simulink model "eAgriBot_V4"  (R2022b)
settings: Solver=ode3  StartTime=0.0  StopTime=t_sim  FixedStep=step_size  RelTol=1e-3
values from neighbouring files (symbols this model uses):
  accel = 0.1*9.81    (= 0.981)    [Run_eAgriBot_V4.m]
  B_tines = 5    [Run_eAgriBot_V4.m]
  brake_bias = 1    [Run_eAgriBot_V4.m]
  c = 6100    [Run_eAgriBot_V4.m]
  decel = 0.15*9.81    (= 1.4715)    [Run_eAgriBot_V4.m]
  decel_begin_dist = total_dist_target    (= 100)    [Run_eAgriBot_V4.m]
  drivetype = 3    [Run_eAgriBot_V4.m]
  effmap = [0.5 0.586 0.723 0.778 0.614 0.604 0.6 0.584 0.709 0.658 0.586 0.688 ... (121 elements, 11x11)]    [EM_effmap_generic.mat]
  end_delay = 4    [Run_eAgriBot_V4.m]
  F_tines = 5    [Run_eAgriBot_V4.m]
  Fb_max = m*g    (= 5101.2)    [Run_eAgriBot_V4.m]
  FT_c_x_rel = l_f    (= 0.645)    [Run_eAgriBot_V4.m]
  FT_c_z_rel = R_u-h_CoG    (= -0.2825)    [Run_eAgriBot_V4.m]
  g = 9.81    [Run_eAgriBot_V4.m]
  gb_eff = 0.98    [Run_eAgriBot_V4.m]
  ground_coh = c*ones(length(ground_points),1)    [Run_eAgriBot_V4.m]
  ground_dens = gamma_s*ones(length(ground_points),1)    [Run_eAgriBot_V4.m]
  ground_height = zeros(length(ground_points),1)    [Run_eAgriBot_V4.m]
  ground_kxy = k_xy*ones(length(ground_points),1)    [Run_eAgriBot_V4.m]
  ground_res = 0.01    [Run_eAgriBot_V4.m]
  Har_back_tip_x_rel = Har_back_top_x_rel+Har_tine_length*cos(Har_angle)    [Run_eAgriBot_V4.m]
  Har_back_tip_z_rel = abs(Hook_z_rel)-h_CoG-Har_tine_depth    [Run_eAgriBot_V4.m]
  Har_back_top_x_rel = -2.0    (= -2)    [Run_eAgriBot_V4.m]
  Har_back_top_z_rel = Har_back_tip_z_rel+Har_tine_length*sin(Har_angle)    [Run_eAgriBot_V4.m]
  Har_front_tip_x_rel = Har_front_top_x_rel+Har_tine_length*cos(Har_angle)    [Run_eAgriBot_V4.m]
  Har_front_tip_z_rel = abs(Hook_z_rel)-h_CoG-Har_tine_depth    [Run_eAgriBot_V4.m]
  Har_front_top_x_rel = -1.2    [Run_eAgriBot_V4.m]
  Har_front_top_z_rel = Har_front_tip_z_rel+Har_tine_length*sin(Har_angle)    [Run_eAgriBot_V4.m]
  Har_tine_length = 0.25    [Run_eAgriBot_V4.m]
  Har_tine_width = 0.02    [Run_eAgriBot_V4.m]
  Har_tire_rad = 0.5842/2    (= 0.2921)    [Run_eAgriBot_V4.m]
  Har_tire_x_rel = -1.5    [Run_eAgriBot_V4.m]
  Har_tire_z_rel = abs(Hook_z_rel)-h_CoG+Har_tire_rad    [Run_eAgriBot_V4.m]
  Hook_x_rel = l_f-l-0.4    (= -1.045)    [Run_eAgriBot_V4.m]
  Hook_z_rel = -0.3    [Run_eAgriBot_V4.m]
  i_front = 17.9542    [Run_eAgriBot_V4.m]
  I_gain = 0.0    (= 0)    [Run_eAgriBot_V4.m]
  i_rear = 17.9542    [Run_eAgriBot_V4.m]
  I_y = 150    [Run_eAgriBot_V4.m]
  I_y_tool = 20    [Run_eAgriBot_V4.m]
  index_init = round(FT_init_exit_x/ground_res)+1    [Run_eAgriBot_V4.m]
  init_CoG_height = h_CoG-0.001    (= 0.599)    [Run_eAgriBot_V4.m]
  init_CoG_v_z = 0    [Run_eAgriBot_V4.m]
  init_omega = 0    [Run_eAgriBot_V4.m]
  init_theta = 0    [Run_eAgriBot_V4.m]
  J_front = J_drive    (= 15)    [Run_eAgriBot_V4.m]
  J_harrow = 1    [Run_eAgriBot_V4.m]
  J_rear = J_drive    (= 15)    [Run_eAgriBot_V4.m]
  k_d = 50e2    (= 5000)    [Run_eAgriBot_V4.m]
  k_d_har = 50e2    (= 5000)    [Run_eAgriBot_V4.m]
  m = 520    [Run_eAgriBot_V4.m]
  m_tool = 200    [Run_eAgriBot_V4.m]
  main_cycle_delay = 5    [Run_eAgriBot_V4.m]
  mu = 0.35    [Run_eAgriBot_V4.m]
  omega_tool_init = 0    [Run_eAgriBot_V4.m]
  P_aux = 200    [Run_eAgriBot_V4.m]
  P_gain = 1.0    (= 1)    [Run_eAgriBot_V4.m]
  pack_Ah = 360    [Battery_data_V5_Kokam_NMC.mat]
  pack_R_charge = [0.00267222222222 0.00267222222222 0.00317777777778 0.00310555555556 0.0026 0.00281666666667 0.00332222222222 0.00353888888889 0.00325 0.00382777777778 0.00382777777778]    [Battery_data_V5_Kokam_NMC.mat]
  pack_R_discharge = [0.00267222222222 0.00267222222222 0.00317777777778 0.00310555555556 0.0026 0.00281666666667 0.00332222222222 0.00353888888889 0.00325 0.00382777777778 0.00382777777778]    [Battery_data_V5_Kokam_NMC.mat]
  pack_VOC = [54.509 52.351 50.895 49.556 48.477 47.645 47.008 46.449 45.825 44.941 44.941]    [Battery_data_V5_Kokam_NMC.mat]
  params2 = [exit_angle reso theta_m_max s_d_tol po]    [Run_eAgriBot_V4.m]
  phi = 26.6    [Run_eAgriBot_V4.m]
  pre_accel = 0.1*9.81    (= 0.981)    [Run_eAgriBot_V4.m]
  pre_decel = 0.15*9.81    (= 1.4715)    [Run_eAgriBot_V4.m]
  pre_decel_begin_dist = pre_dist_target-pre_decel_dist    (= 2.34454218631)    [Run_eAgriBot_V4.m]
  pre_vel = 5    [Run_eAgriBot_V4.m]
  r_front = R_u    (= 0.3175)    [Run_eAgriBot_V4.m]
  r_rear = R_u    (= 0.3175)    [Run_eAgriBot_V4.m]
  rho_t = gamma_s/9.81    (= 1664.01630989)    [Run_eAgriBot_V4.m]
  RT_c_x_rel = l_f-l    (= -0.645)    [Run_eAgriBot_V4.m]
  RT_c_z_rel = R_u-h_CoG    (= -0.2825)    [Run_eAgriBot_V4.m]
  s_init = 3    [Run_eAgriBot_V4.m]
  simu_max_time = cycle_total_time*4    (= 259.930519878)    [Run_eAgriBot_V4.m]
  slip_init = 0    [Run_eAgriBot_V4.m]
  slip_ub = r_rear*1.75    (= 0.555625)    [Run_eAgriBot_V4.m]
  slip_ub_har = Har_tire_rad*1.90    (= 0.55499)    [Run_eAgriBot_V4.m]
  SOC_init = 0.8    [Run_eAgriBot_V4.m]
  SOD = [0 0.1 0.2 0.3 0.4 0.5 0.6 0.7 0.8 0.9 1]    [Battery_data_V5_Kokam_NMC.mat]
  sr_lim_skid = -0.2    [Run_eAgriBot_V4.m]
  sr_lim_slip_f = 0.20-slip_trig    (= 0.18)    [Run_eAgriBot_V4.m]
  sr_lim_slip_r = 0.14-slip_trig    (= 0.12)    [Run_eAgriBot_V4.m]
  step_size = 1e-3    (= 0.001)    [Run_eAgriBot_V4.m]
  T = [80 80 75 70.5882352941 66.6666666667 63.1578947368 60 57.1428571429 54.5454545455 52.1739130435 50 48 ... (49 elements, 49x1)]    [EM_data_V4.mat]    (also in Run_eAgriBot_V4.m = 2*T)
  T_effmap = [0 8 16 24 32 40 48 56 64 72 80]    [EM_effmap_generic.mat]    (also in Run_eAgriBot_V4.m = 2*T_effmap)
  T_multi_r = 1.5    [Run_eAgriBot_V4.m]
  t_params = [c k_c k_phi phi k_xy gamma_s R_u wid c_0 c_1 c_0f c_1f n_0 n_1 k_1 k_2 k_3]    [Run_eAgriBot_V4.m]
  t_params_har = [c k_c k_phi phi k_xy gamma_s Har_tire_rad Har_tire_wid c_0 c_1 c_0f c_1f n_0 n_1 k_1 k_2 k_3]    [Run_eAgriBot_V4.m]
  theta_tool_init = 0    [Run_eAgriBot_V4.m]
  Tine_vz_damping = 0    [Run_eAgriBot_V4.m]
  Tool_x_rel = -1.3    [Run_eAgriBot_V4.m]
  Tool_z_rel = -0.08    [Run_eAgriBot_V4.m]
  v_init = 0    [Run_eAgriBot_V4.m]
  vel_max = 8    [Run_eAgriBot_V4.m]
  w = [0 75 80 85 90 95 100 105 110 115 120 125 ... (49 elements, 49x1)]    [EM_data_V4.mat]
  w_effmap = [0 31.4159265359 62.8318530718 94.2477796077 125.663706144 157.079632679 188.495559215 219.911485751 251.327412287 282.743338823 314.159265359]    [EM_effmap_generic.mat]
libraries: slpidlib x1, simulink x1
(part 4 of 4)

== matlab function eAgriBot_V4/Vehicle dynamics/Ground properties update for tines/MATLAB Function2 ==
  data: kx output; coh output; dens output; index_upd_high input; ground_height output; index_upd_low input; ground_height input; dens input; coh input; kx input; upd_h input; upd_rho input; upd_coh input; upd_kx input
function [kx, coh, dens, ground_height]  = fcn(index_upd_high, index_upd_low, ground_height, dens, coh, kx, upd_h, upd_rho, upd_coh, upd_kx)

for i = index_upd_low:1:index_upd_high
    ground_height(i,1) = upd_h(i,1);
    dens(i,1) = upd_rho(i,1);
    coh(i,1) = upd_coh(i,1);
    kx(i,1) = upd_kx(i,1);
end

== matlab function eAgriBot_V4/Vehicle dynamics/Ground properties update for tines/MATLAB Function3 ==
  data: B_tine_x input; B_tine_z input; ground_height input; dens input; coh input; kx input; ground_res input; upd_B_tine_depth output; upd_dens output; upd_coh output; upd_kx output
function [upd_B_tine_depth, upd_dens, upd_coh, upd_kx] = fcn(B_tine_x, B_tine_z, ground_height, dens, coh, kx, ground_res)

    
    ind_L = max(floor((B_tine_x)/ground_res)+1, 1);
    ind_R = max(ceil((B_tine_x)/ground_res)+1, 1);

    upd_B_tine_depth = B_tine_z-mean(ground_height(ind_L:ind_R));
    upd_dens = mean(dens(ind_L:ind_R));
    upd_coh = mean(coh(ind_L:ind_R));
    upd_kx = mean(kx(ind_L:ind_R));

end

== matlab function eAgriBot_V4/Driver/Main cycle/Deceleration ==
  data: clock input; d_begin_dist input; d input; v_max input; v_target output; cur_dist input; check input; time_d_begin input; check_new output; time_d_begin_new output; end_time input; isover input; end_time_new output; isover_new output
function [v_target, check_new, time_d_begin_new, end_time_new, isover_new] = fcn(clock, d_begin_dist, d, v_max, cur_dist, check, time_d_begin, end_time, isover)
    
    time_d_begin_new = time_d_begin;
    check_new = check;
    end_time_new = end_time;
    isover_new = isover;
    if cur_dist >= d_begin_dist
        if check == 0
            check_new = 1;
            time_d_begin_new = clock;
        end
        v_target = v_max-d*(clock-time_d_begin_new);
    else
        v_target = v_max;
    end

    v_target = max(min(v_target, v_max), 0);

    if check_new == 1 && v_target == 0 && isover == 0
        end_time_new = clock;
        isover_new = 1;
    end

end

== matlab function eAgriBot_V4/Driver/Pre-cycle/Deceleration1 ==
  data: clock input; d_begin_dist input; d input; v_max input; v_target output; cur_dist input; check input; time_d_begin input; check_new output; time_d_begin_new output; end_time input; end_time_new output; isover input; isover_new output
function [v_target, check_new, time_d_begin_new, end_time_new, isover_new] = fcn(clock, d_begin_dist, d, v_max, cur_dist, check, time_d_begin, end_time, isover)
    
    time_d_begin_new = time_d_begin;
    check_new = check;
    end_time_new = end_time;
    isover_new = isover;
    if cur_dist >= d_begin_dist
        if check == 0
            check_new = 1;
            time_d_begin_new = clock;
        end
        v_target = v_max-d*(clock-time_d_begin_new);
    else
        v_target = v_max;
    end

    v_target = max(min(v_target, v_max), 0);

    if check_new == 1 && v_target == 0 && isover == 0
        end_time_new = clock;
        isover_new = 1;
    end

end

== matlab function eAgriBot_V4/Driver/Control/Torque limit based on slip ==
  data: sr_r input; sr_f input; sr_lim_slip_f input; sr_lim_slip_r input; sr_lim_skid input; control input; control_lim_r output; control_lim_f output; drivetype input; T_multi_r input
function [control_lim_r, control_lim_f]= fcn(sr_r, sr_f, sr_lim_slip_f, sr_lim_slip_r, sr_lim_skid, control, drivetype, T_multi_r)
    
    if drivetype < 3
        control = max(min(control, 1), -1);
        control_r = control;
        control_f = control;
    else
        control = max(min(control, 1), -1);
        if control >= 0
            % Optional: increase rear control value and decrease front
            % value such that the difference decreases the higher the
            % control value is.
            % Next three lines commented out by default.
            fac_r = T_multi_r-control*(T_multi_r-1);
            fac_f = (2*control-fac_r*control)/control;
            control_r = control*fac_r;
            control_f = control*fac_f;
%             control_r = control;
%             control_f = control;
        else
            control_r = control;
            control_f = control;
        end
    end

    % Limit control values to +1. This should already be the case and the
    % lines below are just to ensure it.
    control_r = min(control_r, 1);
    control_f = min(control_f, 1);

    % Slip-based limit for rear motor and brake control
    if (sr_r > sr_lim_slip_r) && (control_r > 0)
        sr1 = sr_r;
        control_lim_r = control_r*min(max((((2*sr_lim_slip_r-abs(sr1))/sr_lim_slip_r)^2),0),1);
    elseif (sr_r < sr_lim_skid) && (control_r <= 0)
        sr1 = sr_r;
        control_lim_r = control_r*min(max((((2*abs(sr_lim_skid)-abs(sr1))/abs(sr_lim_skid))^2),0),1);
    else
        control_lim_r = control_r;
    end

    % Slip-based limit for front motor and brake control
    if (sr_f > sr_lim_slip_f) && (control_f > 0)
        sr2 = sr_f;
        control_lim_f = control_f*min(max((((2*sr_lim_slip_f-abs(sr2))/sr_lim_slip_f)^2),0),1);
    elseif (sr_f < sr_lim_skid) && (control_f <= 0)
        sr2 = sr_f;
        control_lim_f = control_f*min(max((((2*abs(sr_lim_skid)-abs(sr2))/abs(sr_lim_skid))^2),0),1);
    else
        control_lim_f = control_f;
    end

    % No front motor throttle if RWD
    if drivetype == 1
        control_lim_f = min(control_lim_f, 0);
    end

    % No rear motor throttle if FWD
    if drivetype == 2
        control_lim_r = min(control_lim_r, 0);
    end

end

== matlab function eAgriBot_V4/Tire model (REAR)/slip_ratio calc ==
  data: r_rear input; v_ms input; RT_vx input; w_tire input; sr output; slip_ub input
function sr = fcn(r_rear, v_ms, RT_vx, w_tire, slip_ub)
    
    ub = slip_ub; % upper bound (when the rotational speed is 1 rad/s)
    lb = 0.1/3.6; % lower bound

    v_ms = max(0, v_ms);

    if abs(v_ms) > ub
        sr = (w_tire*r_rear-RT_vx)/RT_vx;
    elseif abs(v_ms) < lb
        sr = w_tire*r_rear-RT_vx;
    elseif abs(v_ms) <= ub && abs(v_ms) >= lb
        sr = (1/(ub-lb))*(ub-v_ms)*(w_tire*r_rear-RT_vx)+(1/(ub-lb))*(v_ms-lb)*((w_tire*r_rear-RT_vx)/RT_vx);
    else
        sr = 0;
    end

    sr = max(-1, sr);

end

== matlab function eAgriBot_V4/Tire model (FRONT)/Tire force calc1 ==
  data: T output; v_ms input; F_sigma_z output; w_tire_pure input; s_d input; h input; t_params input; params2 input; F_sigma_x output; F_sigma_angle output; F_tau_z output; F_tau_x output; F_tau_angle output; drivetype input
function [T, F_sigma_z, F_sigma_x, F_sigma_angle, F_tau_z, F_tau_x, F_tau_angle]  = fcn(v_ms, w_tire_pure, s_d, h, t_params, params2, drivetype)

    %%

% function [W, F_x, T] = ReeceFuncSim_V1(s_d, h, t_params, params2)
    c = t_params(1); % Pa
    k_c = t_params(2); % 34 default
    k_phi = t_params(3); % 49.68 default
    % n = 0.7;
    phi = t_params(4); % deg
    k_xy = t_params(5); % m
    gamma_s = t_params(6); % N/m^3
    
    R_u = t_params(7); % m (tire radius)
    w = t_params(8); % m (tire width)
    c_0 = t_params(9);
    c_1 = t_params(10);
    c_0f = t_params(11);
    c_1f = t_params(12);
    n_0 = t_params(13);
    n_1 = t_params(14);
    k_1 = t_params(15);
    k_2 = t_params(16);
    k_3 = t_params(17);
    
    exit_angle = params2(1);
    reso = params2(2); % Angle resolution, number of segments per one degree
    
    theta_m_max = params2(3); % Maximum percentage of theta_e allowed for theta_m
    % Allowing this to go too high may result in issues with some
    % calculations outputting complex numbers.
    
    s_d_tol = params2(4);
    
    po = params2(5);
    
    if h < 0
        % Start with defining the angles for theta
        % Then calculate the different values, e.g., sigma_n
        % for each angle.
        % The angle theta starts counter-clockwise from the
        % bottom of the tire (page 3 (267))
        theta_e = min(acos((R_u+max(h,-R_u))/R_u), deg2rad(89));
        theta_b = deg2rad(exit_angle);
        if s_d < -1*s_d_tol
            a = 1/(1+abs(s_d));
        
            d = tan(deg2rad(45)-deg2rad(phi/2));
            
            theta_m = min(2*atan(d./(-a-1)+sqrt(d^2./(-a-1).^2-(-a+1)./(-a-1))), theta_m_max*theta_e);
        elseif s_d >= -1*s_d_tol && s_d <= 0
            a = 1/(1+abs(s_d));
            d = tan(deg2rad(45)-deg2rad(phi/2));
            tm1 = min(2*atan(d./(-a-1)+sqrt(d^2./(-a-1).^2-(-a+1)./(-a-1))), theta_m_max*theta_e);
            tm2 = min((c_0+c_1*abs(s_d)), theta_m_max)*theta_e;
            ft = (1/(s_d_tol)*s_d+1)^po;
            theta_m = (1-ft)*tm1+ft*tm2;
        else
            theta_m = min((c_0+c_1*abs(s_d)), theta_m_max)*theta_e;
        end
        
        angles = linspace(theta_b,theta_e,ceil(rad2deg(theta_e-theta_b)*reso));
        
        l_p = (theta_e-theta_b)*R_u; % Contact arc length
        n = n_0+n_1*abs(s_d);
        b = min(w, l_p);
        
        sigma_n = zeros(length(angles),1);
        W_dtheta = zeros(length(angles),1);
        tau_max = zeros(length(angles),1);
        tau_x = zeros(length(angles),1);
        F_x_dtheta = zeros(length(angles),1);
        T_dtheta = zeros(length(angles),1);
        j_x = zeros(length(angles),1);
        K_v = zeros(length(angles),1);

        F_sigma_dx = zeros(length(angles),1);
        F_sigma_dz = zeros(length(angles),1);
        F_tau_dx = zeros(length(angles),1);
        F_tau_dz = zeros(length(angles),1);

        sigma_theta = zeros(length(angles),1);
        tau_theta = zeros(length(angles),1);
        
        for i = 1:length(angles)
            if angles(i) >= theta_m
                sigma_n(i,1) = (c*k_c+b*gamma_s*k_phi)*(R_u/b)^n*(cos(angles(i))-cos(theta_e))^n;
            else
                sigma_n(i,1) = (c*k_c+b*gamma_s*k_phi)*(R_u/b)^n...
                    *(cos(theta_e-((angles(i)-theta_b)/(theta_m-theta_b)*(theta_e-theta_m)))-cos(theta_e))^n;
            end
            sigma_theta(i,1) = angles(i)*sigma_n(i,1);

            tau_max(i,1) = c+sigma_n(i,1)*tan(deg2rad(phi));
        
            if s_d > 0
                j_x(i,1) = R_u*((theta_e-angles(i))-(1-s_d)*(sin(theta_e)-sin(angles(i))));
            elseif s_d >= -1*s_d_tol && s_d <= 0
                j_x1 = R_u*((theta_e-angles(i))-(1-s_d)*(sin(theta_e)-sin(angles(i))));
                a = 1/(1+abs(s_d));
                K_v(i,1) = a*(((1+abs(s_d))*(sin(theta_e)-sin(theta_m)))/(theta_e-theta_m)-1);
                if angles(i) >= theta_m
                    j_x2 = R_u*((theta_e-angles(i))*(1+K_v(i,1)*(1+abs(s_d)))-(1+abs(s_d))*(sin(theta_e)-sin(angles(i))));
                else
                    j_x2 = R_u*((theta_m-angles(i))-(1+abs(s_d))*(sin(theta_m)-sin(angles(i))));
                end
                ft = (1/(s_d_tol)*s_d+1)^po;
                j_x(i,1) = (1-ft)*j_x2+ft*j_x1;
            else
                a = 1/(1+abs(s_d));
                K_v(i,1) = a*(((1+abs(s_d))*(sin(theta_e)-sin(theta_m)))/(theta_e-theta_m)-1);
                if angles(i) >= theta_m
                    j_x(i,1) = R_u*((theta_e-angles(i))*(1+K_v(i,1)*(1+abs(s_d)))-(1+abs(s_d))*(sin(theta_e)-sin(angles(i))));
                else
                    j_x(i,1) = R_u*((theta_m-angles(i))-(1+abs(s_d))*(sin(theta_m)-sin(angles(i))));
                end
            end
        end
        
        for ii = 1:length(angles)
        
            tau_x(ii,1) = max(min(tau_max(ii,1)*(1-exp(-j_x(ii,1)/k_xy)), abs(tau_max(ii,1))), -1*abs(tau_max(ii,1)));
            tau_theta(ii,1) = angles(ii)*tau_x(ii,1);
        
            W_dtheta(ii,1) = R_u*(sigma_n(ii,1)*cos(angles(ii))+tau_x(ii,1)*sin(angles(ii)));
            F_x_dtheta(ii,1) = R_u*(tau_x(ii,1)*cos(angles(ii))-sigma_n(ii,1)*sin(angles(ii)));
            T_dtheta(ii, 1) = R_u^2*tau_x(ii,1);

            F_sigma_dz(ii,1) = R_u*sigma_n(ii,1)*cos(angles(ii));
            F_sigma_dx(ii,1) = -1*R_u*sigma_n(ii,1)*sin(angles(ii));

            F_tau_dz(ii,1) = R_u*tau_x(ii,1)*sin(angles(ii));
            F_tau_dx(ii,1) = R_u*tau_x(ii,1)*cos(angles(ii));
        end
        
%             W = w*trapz(angles, W_dtheta);
%             F_x = w*trapz(angles, F_x_dtheta);
            T = w*trapz(angles, T_dtheta);

            F_sigma_z = w*trapz(angles, F_sigma_dz);
            F_sigma_x = w*trapz(angles, F_sigma_dx);
            F_sigma_angle = atan(-1*F_sigma_x/F_sigma_z);
            F_tau_z = w*trapz(angles, F_tau_dz);
            F_tau_x = w*trapz(angles, F_tau_dx);
            F_tau_angle = atan(F_tau_z/F_tau_x);

            F_sigma_angle = max(theta_b, min(theta_e, F_sigma_angle));
            F_tau_angle = max(theta_b, min(theta_e, F_tau_angle));

            if v_ms < 0.3/3.6
                F_sigma_angle = max(0, v_ms)*F_sigma_angle*3.6/0.3;
                F_tau_angle = max(0, v_ms)*F_tau_angle*3.6/0.3;
            end
    else
%         W = 0;
%         F_x = 0;
        T = 0;

        F_sigma_z = 0;
        F_sigma_x = 0;
        F_sigma_angle = 0;
        F_tau_z = 0;
        F_tau_x = 0;
        F_tau_angle = 0;
    end

    %%
    
%     if v_ms <= v_low/3.6
%         F_t = (T_axle-J*a_ms/R_u)/R_u;
%         F_t_res = (T_axle-J*a_ms/R_u)/R_u;
%         P = P_lim;
%     elseif (v_ms > v_low/3.6) && (v_up <= 1/3.6)
%     %          F_t = 3.6*(1/(v_up-v_low))*(v_up/3.6-v_ms)*(T_axle-J*a_ms/r)/r+3.6*(1/(v_up-v_low))*(v_ms-v_low/3.6)*(F_z*mu-F_rr);
%          F_t = 3.6*(1/(v_up-v_low))*(v_up/3.6-v_ms)*(T_axle-J*a_ms/R_u)/R_u+3.6*(1/(v_up-v_low))*(v_ms-v_low/3.6)*(F_x);
%          F_t_res = 3.6*(1/(v_up-v_low))*(v_up/3.6-v_ms)*(T_axle-J*a_ms/R_u)/R_u+3.6*(1/(v_up-v_low))*(v_ms-v_low/3.6)*(T/R_u);
%          P = 3.6*(1/(v_up-v_low))*(v_up/3.6-v_ms)*P_lim;
%     else
%         F_t = F_x;
%         F_t_res = T/R_u;
%         P = 0;
%     end

%     F_t = F_x;
    if w_tire_pure <= 0 && v_ms <= 0
%         F_t = 0;
        F_sigma_x = 0;
        F_tau_x = 0;
    end
%     if v_ms <= 0
% %         F_t = max(0, F_t);
%         F_sigma_x = max(0, F_sigma_x);
%         F_tau_x = max(0, F_tau_x);
%     end
    if w_tire_pure <= 0
%         F_t = min(0, F_t);
        F_sigma_x = min(0, F_sigma_x);
        F_tau_x = min(0, F_tau_x);
    end
%     F_t_res = T/R_u;
%     P = 0;
%     P = min(max(P, 0), P_lim);
%     T_Ft_res = F_t_res*R_u+P*(w_tire-v_ms/R_u);
%     T_Ft = F_t*R_u;

    if v_ms < 0
%         F_sigma_x = max(250*abs(v_ms), F_sigma_x);
        F_tau_x = max(500*abs(v_ms), F_tau_x);
    end
    
    if drivetype ~= 2
        F_sigma_x = F_sigma_x*abs(tanh(20*v_ms));
        F_tau_x = F_tau_x*abs(tanh(20*v_ms));
    end

%     if v_ms >= 0 && v_ms < 0.1/3.6 && w_tire_pure <= 0
% %         F_tau_x = F_tau_x-1e5*v_ms;
%         F_tau_x = -1e1*tanh(50*v_ms);
%         F_sigma_x = 0;
%     end

end
